simulink model "T1Linear"  (R2015a)
settings: Solver=ode45  StartTime=0.0  StopTime=100  RelTol=1e-3
undefined symbols (not defined in the file or in its folder): d2wd2t, dw, dwdt
settings Model: Creator=guilh  LastModifiedBy=guilh

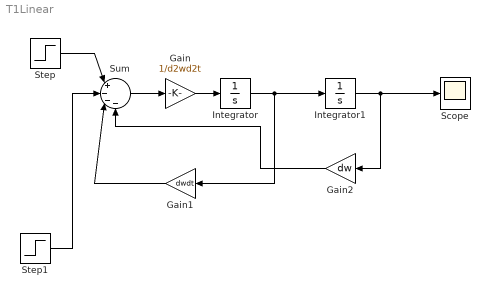
== system T1Linear ==
  Gain : Gain  Gain=1/d2wd2t
  Gain1 : Gain  Gain=dwdt
  Gain2 : Gain  Gain=dw
  Integrator : Integrator
  Integrator1 : Integrator
  Scope : Scope
  Step : Step  Time=0  After=10  SampleTime=0
  Step1 : Step  SampleTime=0
  Sum : Sum  Inputs=|+---
  wires:
  Gain/1 -> Integrator/1
  Sum/1 -> Gain/1
  Integrator/1 -> Gain1/1, Integrator1/1
  Integrator1/1 -> Gain2/1, Scope/1
  Gain2/1 -> Sum/4
  Gain1/1 -> Sum/3
  Step/1 -> Sum/1
  Step1/1 -> Sum/2
